simulink model "red_adelanto_atraso_ao"  (R2020b)
settings: Solver=VariableStepAuto  StartTime=0.0  StopTime=25  MaxStep=1e-4  RelTol=1e-3
values from neighbouring files (symbols this model uses):
  R1 = 10e3    (= 10000)    [atraso_adelanto_c.m]
  R1c = 1/(p1*C1)    (= 20000)    [atraso_adelanto_c.m]
  R2 = R1    (= 10000)    [atraso_adelanto_c.m]
  R2c = 1/(z2*C2)    (= 500000)    [atraso_adelanto_c.m]
  R3 = R1    (= 10000)    [atraso_adelanto_c.m]
  R3c = 1/(z1*C1)-R1c    (= 180000)    [atraso_adelanto_c.m]
  R4 = R1    (= 10000)    [atraso_adelanto_c.m]
  R4c = 1/(p2*C2)-R2c    (= 7500000)    [atraso_adelanto_c.m]
  R5c = 10e3    (= 10000)    [atraso_adelanto_c.m]
  R6c = K*R5c/a    [atraso_adelanto_c.m]
libraries: fl_lib x24, nesl_utility x5, ee_lib x2, simulink x1
settings Model: Creator=cmparedes  LastModifiedBy=Acer
settings DataIOCC: ReturnWorkspaceOutputs=off
settings DebuggingCC: ArithmeticOperatorsInVariantConditions=warning
settings SFSimCC: SimUseLocalCustomCode=off  CustomCodeUndefinedFunction=UseInterfaceOnly
settings RTWCC: RTWUseLocalCustomCode=off

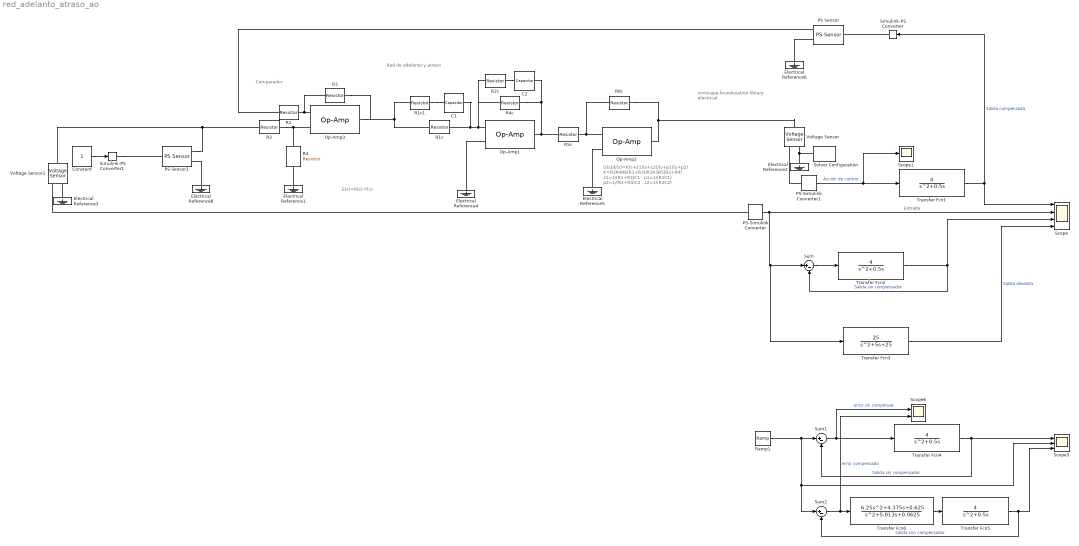
== system red_adelanto_atraso_ao ==
  note: Red de adelanto y atraso
  note: E(s)=R(s)-Y(s)
  note: Comparador
  note: simscape,foundouation library electrical
  note: U(s)/E(s)=K(s+z1)(s+z2)/(s+p1)(s+p2)
      |
      | K=R2R4R6(R1+R3)/R1R3R5(R2+R4)
      | z1=1/(R1+R3)C1  , p1=1/(R1C1)
      | p2=1/(R2+R4)C2  , z2=1/(R2C2)
  C1 : fl_lib/Electrical/Electrical Elements/Capacitor  c=C1 F  r=1e-6 Ohm  g=0 1/Ohm  i_specify=off  i_priority=None  i=0 A  i_nominal_specify=off  i_nominal_unit=A  i_nominal_value=1  v_specify=off  v_priority=None  v=0 V  v_nominal_specify=off  v_nominal_unit=V  v_nominal_value=1  vc_specify=off  vc_priority=High  vc=0 V  vc_nominal_specify=off  vc_nominal_unit=V  vc_nominal_value=1
  C2 : fl_lib/Electrical/Electrical Elements/Capacitor  c=C2 F  r=1e-6 Ohm  g=0 1/Ohm  i_specify=off  i_priority=None  i=0 A  i_nominal_specify=off  i_nominal_unit=A  i_nominal_value=1  v_specify=off  v_priority=None  v=0 V  v_nominal_specify=off  v_nominal_unit=V  v_nominal_value=1  vc_specify=off  vc_priority=High  vc=0 V  vc_nominal_specify=off  vc_nominal_unit=V  vc_nominal_value=1
  Constant : Constant  VectorParams1D=off  SampleTime=-1
  Electrical Reference{1..6,8} (7 alike) : fl_lib/Electrical/Electrical Elements/Electrical Reference
  Op-Amp1 : fl_lib/Electrical/Electrical Elements/Op-Amp  outI_specify=off  outI_priority=None  outI=0 A  outI_nominal_specify=off  outI_nominal_unit=A  outI_nominal_value=1
  Op-Amp2 : fl_lib/Electrical/Electrical Elements/Op-Amp  outI_specify=off  outI_priority=None  outI=0 A  outI_nominal_specify=off  outI_nominal_unit=A  outI_nominal_value=1
  Op-Amp3 : fl_lib/Electrical/Electrical Elements/Op-Amp  outI_specify=off  outI_priority=None  outI=0 A  outI_nominal_specify=off  outI_nominal_unit=A  outI_nominal_value=1
  PS Sensor : ee_lib/Sensors & Transducers/PS Sensor  op_type=1  A=1  B=0  Ymax=inf  Ymin=-inf
      settings: SourceProductBaseCode=PS  InternalSimscapePortConfiguration="{\"Bottom\":[],\"Left\":[{\"id\":\"U\",\"label\":\"U\",\"type\":\"input\"}],\"Right\":[{\"id\":\"p\",\"label\":\"+\",\"type\":\"foundation.electrical.electrical\"},{\"id\":\"n\",\"label\":\"-\",\"type\":\"foundation.electrical.electrical\"}],\"Top\":[]}"
  PS Sensor1 : ee_lib/Sensors & Transducers/PS Sensor  op_type=1  A=1  B=0  Ymax=inf  Ymin=-inf
      settings: SourceProductBaseCode=PS  InternalSimscapePortConfiguration="{\"Bottom\":[],\"Left\":[{\"id\":\"U\",\"label\":\"U\",\"type\":\"input\"}],\"Right\":[{\"id\":\"p\",\"label\":\"+\",\"type\":\"foundation.electrical.electrical\"},{\"id\":\"n\",\"label\":\"-\",\"type\":\"foundation.electrical.electrical\"}],\"Top\":[]}"
  PS-Simulink Converter : nesl_utility/PS-Simulink Converter  PhysicalDomain=network_engine_domain  SubClassName=ps_output  LeftPortType=input  RightPortType=output  PseudoPeriodic=off  Frequencies=[]  Unit=1  AffineConversion=off
  PS-Simulink Converter1 : nesl_utility/PS-Simulink Converter  PhysicalDomain=network_engine_domain  SubClassName=ps_output  LeftPortType=input  RightPortType=output  PseudoPeriodic=off  Frequencies=[]  Unit=1  AffineConversion=off
  R1 : fl_lib/Electrical/Electrical Elements/Resistor  R=R1 Ohm  i_specify=off  i_priority=None  i=0 A  i_nominal_specify=off  i_nominal_unit=A  i_nominal_value=1  v_specify=off  v_priority=None  v=0 V  v_nominal_specify=off  v_nominal_unit=V  v_nominal_value=1
  R1c : fl_lib/Electrical/Electrical Elements/Resistor  R=R3c Ohm  i_specify=off  i_priority=None  i=0 A  i_nominal_specify=off  i_nominal_unit=A  i_nominal_value=1  v_specify=off  v_priority=None  v=0 V  v_nominal_specify=off  v_nominal_unit=V  v_nominal_value=1
  R1c1 : fl_lib/Electrical/Electrical Elements/Resistor  R=R1c Ohm  i_specify=off  i_priority=None  i=0 A  i_nominal_specify=off  i_nominal_unit=A  i_nominal_value=1  v_specify=off  v_priority=None  v=0 V  v_nominal_specify=off  v_nominal_unit=V  v_nominal_value=1
  R2 : fl_lib/Electrical/Electrical Elements/Resistor  R=R2 Ohm  i_specify=off  i_priority=None  i=0 A  i_nominal_specify=off  i_nominal_unit=A  i_nominal_value=1  v_specify=off  v_priority=None  v=0 V  v_nominal_specify=off  v_nominal_unit=V  v_nominal_value=1
  R2c : fl_lib/Electrical/Electrical Elements/Resistor  R=R2c Ohm  i_specify=off  i_priority=None  i=0 A  i_nominal_specify=off  i_nominal_unit=A  i_nominal_value=1  v_specify=off  v_priority=None  v=0 V  v_nominal_specify=off  v_nominal_unit=V  v_nominal_value=1
  R3 : fl_lib/Electrical/Electrical Elements/Resistor  R=R3 Ohm  i_specify=off  i_priority=None  i=0 A  i_nominal_specify=off  i_nominal_unit=A  i_nominal_value=1  v_specify=off  v_priority=None  v=0 V  v_nominal_specify=off  v_nominal_unit=V  v_nominal_value=1
  R4 : fl_lib/Electrical/Electrical Elements/Resistor  R=R4 Ohm  i_specify=off  i_priority=None  i=0 A  i_nominal_specify=off  i_nominal_unit=A  i_nominal_value=1  v_specify=off  v_priority=None  v=0 V  v_nominal_specify=off  v_nominal_unit=V  v_nominal_value=1
  R4c : fl_lib/Electrical/Electrical Elements/Resistor  R=R4c Ohm  i_specify=off  i_priority=None  i=0 A  i_nominal_specify=off  i_nominal_unit=A  i_nominal_value=1  v_specify=off  v_priority=None  v=0 V  v_nominal_specify=off  v_nominal_unit=V  v_nominal_value=1
  R5c : fl_lib/Electrical/Electrical Elements/Resistor  R=R5c Ohm  i_specify=off  i_priority=None  i=0 A  i_nominal_specify=off  i_nominal_unit=A  i_nominal_value=1  v_specify=off  v_priority=None  v=0 V  v_nominal_specify=off  v_nominal_unit=V  v_nominal_value=1
  R6c : fl_lib/Electrical/Electrical Elements/Resistor  R=R6c Ohm  i_specify=off  i_priority=None  i=0 A  i_nominal_specify=off  i_nominal_unit=A  i_nominal_value=1  v_specify=off  v_priority=None  v=0 V  v_nominal_specify=off  v_nominal_unit=V  v_nominal_value=1
  Ramp1 : simulink/Sources/Ramp  slope=1  start=0  InitialOutput=0
  Scope : Scope  NumInputPorts=4
  Scope1 : Scope
  Scope3 : Scope  NumInputPorts=3
  Scope6 : Scope  NumInputPorts=2
  Simulink-PS Converter : nesl_utility/Simulink-PS Converter  PhysicalDomain=network_engine_domain  SubClassName=ps_input  LeftPortType=input  RightPortType=output  PseudoPeriodic=off  Frequencies=[]  NoiseDistribution=none  NoiseParameters=[]  Unit=1  AffineConversion=off  FilteringAndDerivatives=provide  SimscapeFilterOrder=1  InputFilterTimeConstant=0.001  UdotUserProvided=0
  Simulink-PS Converter1 : nesl_utility/Simulink-PS Converter  PhysicalDomain=network_engine_domain  SubClassName=ps_input  LeftPortType=input  RightPortType=output  PseudoPeriodic=off  Frequencies=[]  NoiseDistribution=none  NoiseParameters=[]  Unit=1  AffineConversion=off  FilteringAndDerivatives=provide  SimscapeFilterOrder=1  InputFilterTimeConstant=0.001  UdotUserProvided=0
  Solver Configuration : nesl_utility/Solver Configuration  PhysicalDomain=network_engine_domain  SubClassName=solver  LeftPortType=input  RightPortType=generic  Tones=[]  Harmonics=[]  SimulateNoise=off  Profile=off  UseLocalSampling=off  EnableSwitchedLinearOptims=on  FrequencyDomain=off  UseCCode=off  RelTol=0.001  AbsTol=1e-06  MinStep=1e-09  ToWorkspace=off  RevertToSquareIcSolve=off  NumHomotopyIterations=100  PhasorMode=off  PhasorModeNumHarmonics=1  DoDC=off  ResidualTolerance=1e-09  UseLocalSolver=off  LocalSolverChoice=NE_BACKWARD_EULER_ADVANCER  LocalSolverSampleTime=0.001  DoFixedCost=off  MaxNonlinIter=3  MaxModeIter=2  ComputeImpulses=off  ImpulseIterations=2  LinearAlgebra=Sparse  EquationFormulation=NE_TIME_EF  DelaysMemoryBudget=1024  AutomaticFiltering=on  FilteringTimeConstant=0.001  PartitionStorageMethod=AS_NEEDED  PartitionMemoryBudget=1024  PartitionMethod=FAST
  Sum : Sum  Inputs=|+-
  Sum1 : Sum  Inputs=|+-
  Sum2 : Sum  Inputs=|+-
  Transfer Fcn{1..2,4..5} (4 alike) : TransferFcn  Numerator=4  Denominator=[1 0.5 0]
  Transfer Fcn3 : TransferFcn  Numerator=25  Denominator=[1 5 25]
  Transfer Fcn6 : TransferFcn  Numerator=[6.25 4.375 0.625]  Denominator=[1 5.013 0.0625]
  Voltage Sensor : fl_lib/Electrical/Electrical Sensors/Voltage Sensor
  Voltage Sensor1 : fl_lib/Electrical/Electrical Sensors/Voltage Sensor
  wires:
  PS-Simulink Converter1/1 -> Transfer Fcn1/1, Scope1/1  "Acción de control"
  PS-Simulink Converter/1 -> Transfer Fcn3/1, Sum/1, Scope/2  "Entrada"
  Transfer Fcn1/1 -> Scope/1, Simulink-PS Converter/1  "Salida compensada"
  Sum/1 -> Transfer Fcn2/1
  Transfer Fcn2/1 -> Sum/2, Scope/3  "Salida sin compensador"
  Constant/1 -> Simulink-PS Converter1/1
  Transfer Fcn3/1 -> Scope/4  "Salida deseada"
  Sum1/1 -> Scope6/1, Transfer Fcn4/1  "error sin compensar"
  Ramp1/1 -> Sum1/1, Sum2/1, Scope3/2
  Transfer Fcn4/1 -> Scope3/1, Sum1/2  "Salida sin compensador"
  Transfer Fcn5/1 -> Sum2/2, Scope3/3  "Salida con compensador"
  Sum2/1 -> Scope6/2, Transfer Fcn6/1  "error compensado"
  Transfer Fcn6/1 -> Transfer Fcn5/1
  connections:
  Electrical Reference2/LConn1 -- Solver Configuration/RConn1 -- Voltage Sensor/RConn2
  PS-Simulink Converter1/LConn1 -- Voltage Sensor/RConn1
  PS-Simulink Converter/LConn1 -- Voltage Sensor1/RConn1
  R2/RConn1 -- R4/RConn1 -- Op-Amp3/LConn1
  Electrical Reference1/LConn1 -- R4/LConn1
  R1/RConn1 -- R3/LConn1 -- Op-Amp3/LConn2
  Voltage Sensor1/LConn1 -- PS Sensor1/RConn1 -- R2/LConn1
  Electrical Reference3/LConn1 -- Voltage Sensor1/RConn2
  Op-Amp1/LConn2 -- R2c/LConn1 -- R4c/LConn1 -- C1/RConn1 -- R1c/RConn1
  R4c/RConn1 -- C2/RConn1 -- R5c/LConn1 -- Op-Amp1/RConn1
  Electrical Reference4/LConn1 -- Op-Amp1/LConn1
  R3/RConn1 -- Op-Amp3/RConn1 -- R1c1/LConn1 -- R1c/LConn1
  R5c/RConn1 -- R6c/LConn1 -- Op-Amp2/LConn2
  R6c/RConn1 -- Voltage Sensor/LConn1 -- Op-Amp2/RConn1
  Electrical Reference5/LConn1 -- Op-Amp2/LConn1
  PS Sensor/RConn1 -- R1/LConn1
  Simulink-PS Converter/RConn1 -- PS Sensor/LConn1
  PS Sensor/RConn2 -- Electrical Reference6/LConn1
  Simulink-PS Converter1/RConn1 -- PS Sensor1/LConn1
  Electrical Reference8/LConn1 -- PS Sensor1/RConn2
  R1c1/RConn1 -- C1/LConn1
  R2c/RConn1 -- C2/LConn1
